simulink model "Motor_Control_position"  (R2020b)
settings: Solver=VariableStepAuto  StartTime=0.0  StopTime=10.0  RelTol=1e-3
values from neighbouring files (symbols this model uses):
  b = 3.5077E-6    [motor_parameters.sldd]
  J = 3.2284E-6    [motor_parameters.sldd]
  Ke = 0.0274    [motor_parameters.sldd]
  Kt = 0.0274    [motor_parameters.sldd]
  L = 2.75E-6    [motor_parameters.sldd]
  R = 4.0    [motor_parameters.sldd]
settings Model: Creator=shivanshu shukla  LastModifiedBy=shivanshu shukla

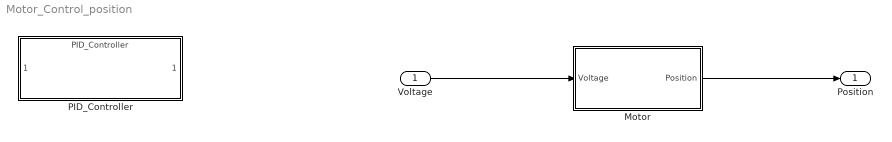
== system Motor_Control_position ==
  Voltage : Inport
  Motor : Subsystem
  PID_Controller : ModelReference  ModelNameDialog=PID_Controller  SimulationMode=Normal  ModelReferenceVersion=1.2
  Position : Outport
  wires:
  Voltage/1 -> Motor/1(Voltage)
  Motor/1(Position) -> Position/1

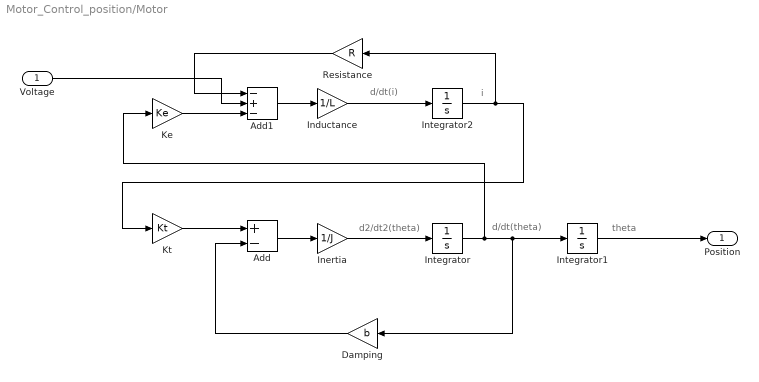
== system Motor_Control_position/Motor ==
  note: d/dt(i)
  note: d/dt(theta)
  note: theta
  note: d2/dt2(theta)
  note: i
  Voltage : Inport
  Add : Sum  Inputs=+-
  Add1 : Sum  Inputs=-+-
  Damping : Gain  Gain=b
  Inductance : Gain  Gain=1/L
  Inertia : Gain  Gain=1/J
  Integrator : Integrator
  Integrator1 : Integrator
  Integrator2 : Integrator
  Ke : Gain  Gain=Ke
  Kt : Gain  Gain=Kt
  Resistance : Gain  Gain=R
  Position : Outport
  wires:
  Integrator2/1 -> Resistance/1, Kt/1
  Add1/1 -> Inductance/1
  Integrator1/1 -> Position/1
  Damping/1 -> Add/2
  Inductance/1 -> Integrator2/1
  Integrator/1 -> Ke/1, Damping/1, Integrator1/1
  Resistance/1 -> Add1/1
  Kt/1 -> Add/1
  Voltage/1 -> Add1/2
  Inertia/1 -> Integrator/1
  Ke/1 -> Add1/3
  Add/1 -> Inertia/1
